simulink model "flc_acoplado"  (R2018b)
settings: Solver=VariableStepAuto  StartTime=0.0  StopTime=50  RelTol=1e-3
libraries: fuzblock x2
settings Model: Creator=root  LastModifiedBy=root

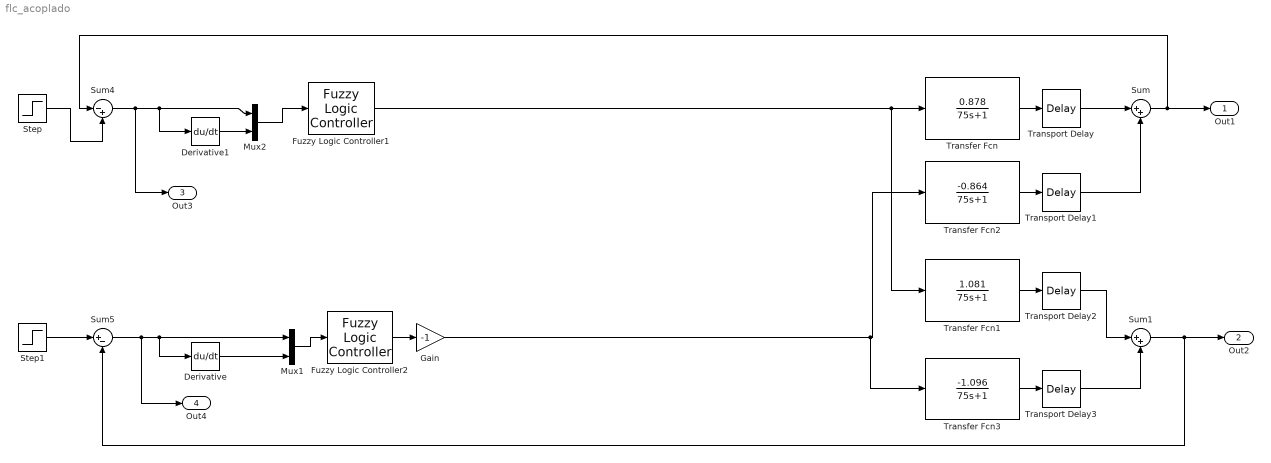
== system flc_acoplado ==
  Derivative : Derivative
  Derivative1 : Derivative
  Fuzzy Logic Controller1 : fuzblock/Fuzzy Logic  Controller  FIS=flc1  OutputSampleNumber=101  DataType=double  FuzzifiedInputs=off  RuleFiringStrengths=off  RuleOutputs=off  AggregatedOutputs=off  SimulateUsing=Interpreted execution  OutOfRangeInputValueMessage=warning  NoRuleFiredMessage=warning  EmptyOutputFuzzySetMessage=warning
  Fuzzy Logic Controller2 : fuzblock/Fuzzy Logic  Controller  FIS=flc2  OutputSampleNumber=101  DataType=double  FuzzifiedInputs=off  RuleFiringStrengths=off  RuleOutputs=off  AggregatedOutputs=off  SimulateUsing=Interpreted execution  OutOfRangeInputValueMessage=warning  NoRuleFiredMessage=warning  EmptyOutputFuzzySetMessage=warning
  Gain : Gain  Gain=-1
  Mux1 : Mux  Inputs=2
  Mux2 : Mux  Inputs=2
  Step : Step  SampleTime=0
  Step1 : Step  After=0  SampleTime=0
  Sum : Sum  Inputs=|++
  Sum1 : Sum  Inputs=|++
  Sum4 : Sum  Inputs=|-+
  Sum5 : Sum  Inputs=|+-
  Transfer Fcn : TransferFcn  Numerator=[0.878]  Denominator=[75 1]
  Transfer Fcn1 : TransferFcn  Numerator=[1.081]  Denominator=[75 1]
  Transfer Fcn2 : TransferFcn  Numerator=[-0.864]  Denominator=[75 1]
  Transfer Fcn3 : TransferFcn  Numerator=[-1.096]  Denominator=[75 1]
  Transport Delay{,1..3} (4 alike) : TransportDelay
  Out1 : Outport  SignalName=y1
  Out2 : Outport  Port=2  SignalName=y2
  Out3 : Outport  Port=3  SignalName=y1
  Out4 : Outport  Port=4  SignalName=y1
  wires:
  Transfer Fcn/1 -> Transport Delay/1
  Fuzzy Logic Controller2/1 -> Gain/1
  Gain/1 -> Transfer Fcn3/1, Transfer Fcn2/1
  Sum4/1 -> Out3/1, Derivative1/1, Mux2/1
  Step1/1 -> Sum5/1
  Sum5/1 -> Out4/1, Derivative/1, Mux1/1
  Mux1/1 -> Fuzzy Logic Controller2/1
  Derivative1/1 -> Mux2/2
  Transport Delay/1 -> Sum/1
  Transport Delay3/1 -> Sum1/2
  Transfer Fcn1/1 -> Transport Delay2/1
  Step/1 -> Sum4/2
  Transport Delay2/1 -> Sum1/1
  Transfer Fcn3/1 -> Transport Delay3/1
  Fuzzy Logic Controller1/1 -> Transfer Fcn1/1, Transfer Fcn/1
  Transfer Fcn2/1 -> Transport Delay1/1
  Derivative/1 -> Mux1/2
  Mux2/1 -> Fuzzy Logic Controller1/1
  Transport Delay1/1 -> Sum/2
  Sum1/1 -> Sum5/2, Out2/1
  Sum/1 -> Sum4/1, Out1/1
